simulink model "DCMGHILS"  (Simulink 7.9)
settings: Solver=ode4  StartTime=0.0  StopTime=inf  FixedStep=.1  RelTol=1e-3
StartFcn:
  | h=add_exec_event_listener('DCMGHILS/GUIScope','PostOutputs',@GUIScope);
values from neighbouring files (symbols this model uses):
  Manual = evalin('base','Manual')    [DCMicrogrid2.m]
libraries: simulink x24, opclib x3
settings Model: Creator=Don  LastModifiedBy=Microgrid_Project
settings DebuggingCC: FcnCallInpInsideContextMsg=Use local settings
settings GRTTargetCC: CombineOutputUpdateFcns=off  GRTInterface=on

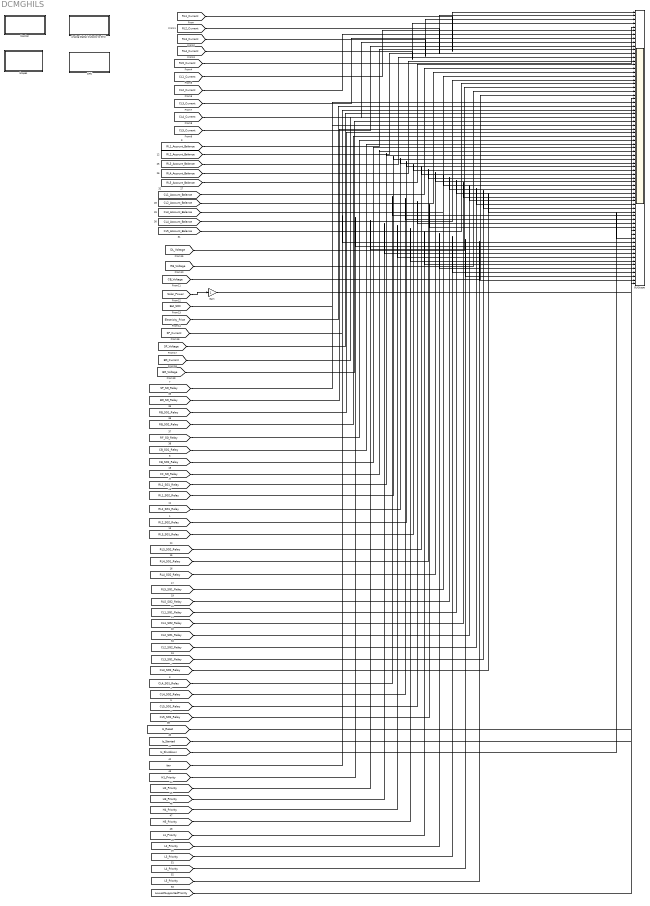
== system DCMGHILS ==
  Analog Digital Outputs to Grid : Subsystem
  GUIScope : Scope  NumInputPorts=73
      settings: YMin=-5~-5~-5~-5~-5~-5~-5~-5~-5~-5~-5~-5~-5~-5~-5~-5~-5~-5~-5~-5~-5~-5~-5~-5~-5~-5~-5~-5~-5~-5~-5~-5~-5~-5~-5~-5~-5~-5~-5~-5~-5~-5~-5~-5~-5~-5~-5~-5~-5~-5~-5~-5~-5~-5~-5~-5~-5~-5~-5~-5~-5~-5~-5~-5~-5~-5~-5~-5~-5~-5~-5~-5~-5  YMax=5~5~5~5~5~5~5~5~5~5~5~5~5~5~5~5~5~5~5~5~5~5~5~5~5~5~5~5~5~5~5~5~5~5~5~5~5~5~5~5~5~5~5~5~5~5~5~5~5~5~5~5~5~5~5~5~5~5~5~5~5~5~5~5~5~5~5~5~5~5~5~5~5  MaxDataPoints=10  SampleInput=on  SampleTime=.1
  Gain : Gain
  Monitor : Subsystem
  OPC : Subsystem
  Scopes : Subsystem
  wires:
  [Solar_Power] -> Gain/1
  [RL1_Current] -> GUIScope/1
  [RL2_Current] -> GUIScope/2
  [RL3_Current] -> GUIScope/3
  [RL4_Current] -> GUIScope/4
  [RL5_Current] -> GUIScope/5
  [CL1_Current] -> GUIScope/6
  [CL2_Current] -> GUIScope/7
  Gain/1 -> GUIScope/24
  [CL3_Current] -> GUIScope/8
  [CL4_Current] -> GUIScope/9
  [CL5_Current] -> GUIScope/10
  [RL1_Account_Balance] -> GUIScope/11
  [RL2_Account_Balance] -> GUIScope/12
  [RL3_Account_Balance] -> GUIScope/13
  [RL4_Account_Balance] -> GUIScope/14
  [RL5_Account_Balance] -> GUIScope/15
  [CL1_Account_Balance] -> GUIScope/16
  [CL2_Account_Balance] -> GUIScope/17
  [CL3_Account_Balance] -> GUIScope/18
  [CL4_Account_Balance] -> GUIScope/19
  [CL5_Account_Balance] -> GUIScope/20
  [DL_Voltage] -> GUIScope/21
  [RB_Voltage] -> GUIScope/22
  [CB_Voltage] -> GUIScope/23
  [Bat_SOC] -> GUIScope/25
  [Electricity_Price] -> GUIScope/26
  [SP_Current] -> GUIScope/27
  [SP_Voltage] -> GUIScope/28
  [BG_Current] -> GUIScope/29
  [BG_Voltage] -> GUIScope/30
  [SP_SG_Relay] -> GUIScope/31
  [BG_SG_Relay] -> GUIScope/32
  [RB_SG1_Relay] -> GUIScope/33
  [RB_SG2_Relay] -> GUIScope/34
  [RF_SG_Relay] -> GUIScope/35
  [CB_SG1_Relay] -> GUIScope/36
  [CB_SG2_Relay] -> GUIScope/37
  [CF_SG_Relay] -> GUIScope/38
  [RL1_SG1_Relay] -> GUIScope/39
  [RL1_SG2_Relay] -> GUIScope/40
  [RL2_SG1_Relay] -> GUIScope/41
  [RL2_SG2_Relay] -> GUIScope/42
  [RL3_SG1_Relay] -> GUIScope/43
  [RL3_SG2_Relay] -> GUIScope/44
  [RL4_SG1_Relay] -> GUIScope/45
  [RL4_SG2_Relay] -> GUIScope/46
  [RL5_SG1_Relay] -> GUIScope/47
  [RL5_SG2_Relay] -> GUIScope/48
  [CL1_SG1_Relay] -> GUIScope/49
  [CL1_SG2_Relay] -> GUIScope/50
  [CL2_SG1_Relay] -> GUIScope/51
  [CL2_SG2_Relay] -> GUIScope/52
  [CL3_SG1_Relay] -> GUIScope/53
  [CL3_SG2_Relay] -> GUIScope/54
  [CL4_SG1_Relay] -> GUIScope/55
  [CL4_SG2_Relay] -> GUIScope/56
  [CL5_SG1_Relay] -> GUIScope/57
  [CL5_SG2_Relay] -> GUIScope/58
  [iter] -> GUIScope/62
  [H1_Priority] -> GUIScope/63
  [H2_Priority] -> GUIScope/64
  [H3_Priority] -> GUIScope/65
  [H4_Priority] -> GUIScope/66
  [H5_Priority] -> GUIScope/67
  [L1_Priority] -> GUIScope/68
  [L2_Priority] -> GUIScope/69
  [L3_Priority] -> GUIScope/70
  [L4_Priority] -> GUIScope/71
  [L5_Priority] -> GUIScope/72
  [Is_Reset] -> GUIScope/59
  [Is_Started] -> GUIScope/60
  [Is_Shutdown] -> GUIScope/61
  [LowestSupportedPriority] -> GUIScope/73

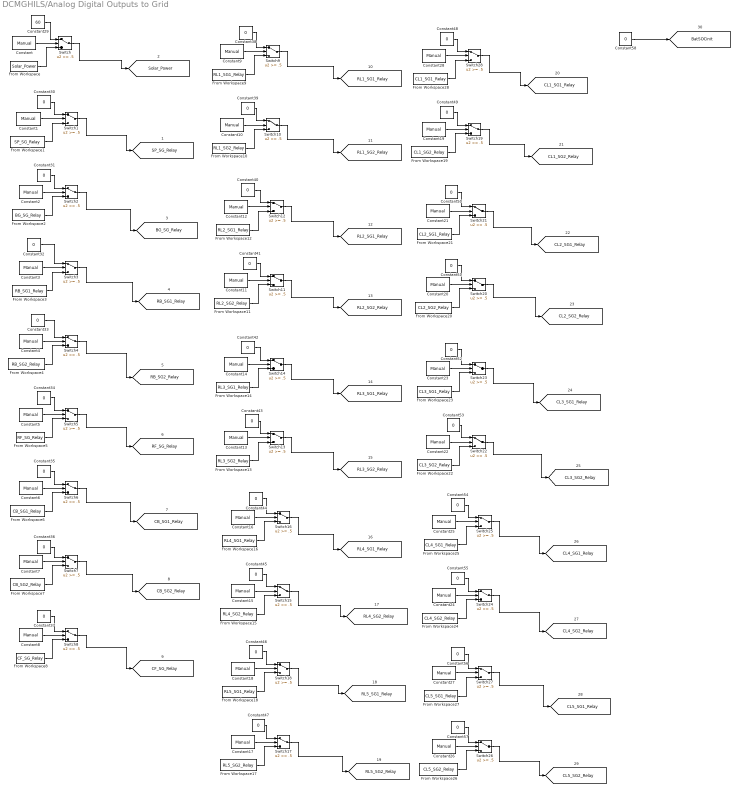
== system DCMGHILS/Analog Digital Outputs to Grid ==
  Constant{,1..28} (29 alike) : Constant  Value=Manual
  Constant29 : Constant  Value=60
  Constant{30..58} (29 alike) : Constant  Value=0
  From Workspace : FromWorkspace  VariableName=Solar_Power  SampleTime=0  Interpolate=off  OutputAfterFinalValue=Holding final value
  From Workspace1 : FromWorkspace  VariableName=SP_SG_Relay  SampleTime=0  Interpolate=off  OutputAfterFinalValue=Holding final value
  From Workspace10 : FromWorkspace  VariableName=RL1_SG2_Relay  SampleTime=0  Interpolate=off  OutputAfterFinalValue=Holding final value
  From Workspace11 : FromWorkspace  VariableName=RL2_SG2_Relay  SampleTime=0  Interpolate=off  OutputAfterFinalValue=Holding final value
  From Workspace12 : FromWorkspace  VariableName=RL2_SG1_Relay  SampleTime=0  Interpolate=off  OutputAfterFinalValue=Holding final value
  From Workspace13 : FromWorkspace  VariableName=RL3_SG2_Relay  SampleTime=0  Interpolate=off  OutputAfterFinalValue=Holding final value
  From Workspace14 : FromWorkspace  VariableName=RL3_SG1_Relay  SampleTime=0  Interpolate=off  OutputAfterFinalValue=Holding final value
  From Workspace15 : FromWorkspace  VariableName=RL4_SG2_Relay  SampleTime=0  Interpolate=off  OutputAfterFinalValue=Holding final value
  From Workspace16 : FromWorkspace  VariableName=RL4_SG1_Relay  SampleTime=0  Interpolate=off  OutputAfterFinalValue=Holding final value
  From Workspace17 : FromWorkspace  VariableName=RL5_SG2_Relay  SampleTime=0  Interpolate=off  OutputAfterFinalValue=Holding final value
  From Workspace18 : FromWorkspace  VariableName=RL5_SG1_Relay  SampleTime=0  Interpolate=off  OutputAfterFinalValue=Holding final value
  From Workspace19 : FromWorkspace  VariableName=CL1_SG2_Relay  SampleTime=0  Interpolate=off  OutputAfterFinalValue=Holding final value
  From Workspace2 : FromWorkspace  VariableName=BG_SG_Relay  SampleTime=0  Interpolate=off  OutputAfterFinalValue=Holding final value
  From Workspace20 : FromWorkspace  VariableName=CL2_SG2_Relay  SampleTime=0  Interpolate=off  OutputAfterFinalValue=Holding final value
  From Workspace21 : FromWorkspace  VariableName=CL2_SG1_Relay  SampleTime=0  Interpolate=off  OutputAfterFinalValue=Holding final value
  From Workspace22 : FromWorkspace  VariableName=CL3_SG2_Relay  SampleTime=0  Interpolate=off  OutputAfterFinalValue=Holding final value
  From Workspace23 : FromWorkspace  VariableName=CL3_SG1_Relay  SampleTime=0  Interpolate=off  OutputAfterFinalValue=Holding final value
  From Workspace24 : FromWorkspace  VariableName=CL4_SG2_Relay  SampleTime=0  Interpolate=off  OutputAfterFinalValue=Holding final value
  From Workspace25 : FromWorkspace  VariableName=CL4_SG1_Relay  SampleTime=0  Interpolate=off  OutputAfterFinalValue=Holding final value
  From Workspace26 : FromWorkspace  VariableName=CL5_SG2_Relay  SampleTime=0  Interpolate=off  OutputAfterFinalValue=Holding final value
  From Workspace27 : FromWorkspace  VariableName=CL5_SG1_Relay  SampleTime=0  Interpolate=off  OutputAfterFinalValue=Holding final value
  From Workspace28 : FromWorkspace  VariableName=CL1_SG1_Relay  SampleTime=0  Interpolate=off  OutputAfterFinalValue=Holding final value
  From Workspace3 : FromWorkspace  VariableName=RB_SG1_Relay  SampleTime=0  Interpolate=off  OutputAfterFinalValue=Holding final value
  From Workspace4 : FromWorkspace  VariableName=RB_SG2_Relay  SampleTime=0  Interpolate=off  OutputAfterFinalValue=Holding final value
  From Workspace5 : FromWorkspace  VariableName=RF_SG_Relay  SampleTime=0  Interpolate=off  OutputAfterFinalValue=Holding final value
  From Workspace6 : FromWorkspace  VariableName=CB_SG1_Relay  SampleTime=0  Interpolate=off  OutputAfterFinalValue=Holding final value
  From Workspace7 : FromWorkspace  VariableName=CB_SG2_Relay  SampleTime=0  Interpolate=off  OutputAfterFinalValue=Holding final value
  From Workspace8 : FromWorkspace  VariableName=CF_SG_Relay  SampleTime=0  Interpolate=off  OutputAfterFinalValue=Holding final value
  From Workspace9 : FromWorkspace  VariableName=RL1_SG1_Relay  SampleTime=0  Interpolate=off  OutputAfterFinalValue=Holding final value
  Switch{,1..28} (29 alike) : Switch  Threshold=.5
  tag scope: BG_SG_Relay=global, BatSOCinit=global, CB_SG1_Relay=global, CB_SG2_Relay=global, CF_SG_Relay=global, CL1_SG1_Relay=global, CL1_SG2_Relay=global, CL2_SG1_Relay=global, CL2_SG2_Relay=global, CL3_SG1_Relay=global, CL3_SG2_Relay=global, CL4_SG1_Relay=global, CL4_SG2_Relay=global, CL5_SG1_Relay=global, CL5_SG2_Relay=global, RB_SG1_Relay=global, RB_SG2_Relay=global, RF_SG_Relay=global, RL1_SG1_Relay=global, RL1_SG2_Relay=global, RL2_SG1_Relay=global, RL2_SG2_Relay=global, RL3_SG1_Relay=global, RL3_SG2_Relay=global, RL4_SG1_Relay=global, RL4_SG2_Relay=global, RL5_SG1_Relay=global, RL5_SG2_Relay=global, SP_SG_Relay=global, Solar_Power=global
  wires:
  Constant/1 -> Switch/2
  From Workspace/1 -> Switch/3
  Constant29/1 -> Switch/1
  Switch/1 -> [Solar_Power]
  Constant1/1 -> Switch1/2
  From Workspace1/1 -> Switch1/3
  Constant30/1 -> Switch1/1
  Switch1/1 -> [SP_SG_Relay]
  Constant2/1 -> Switch2/2
  From Workspace2/1 -> Switch2/3
  Constant31/1 -> Switch2/1
  Switch2/1 -> [BG_SG_Relay]
  Constant3/1 -> Switch3/2
  From Workspace3/1 -> Switch3/3
  Constant32/1 -> Switch3/1
  Switch3/1 -> [RB_SG1_Relay]
  Constant4/1 -> Switch4/2
  From Workspace4/1 -> Switch4/3
  Constant33/1 -> Switch4/1
  Switch4/1 -> [RB_SG2_Relay]
  Constant5/1 -> Switch5/2
  From Workspace5/1 -> Switch5/3
  Constant34/1 -> Switch5/1
  Switch5/1 -> [RF_SG_Relay]
  Constant6/1 -> Switch6/2
  From Workspace6/1 -> Switch6/3
  Constant35/1 -> Switch6/1
  Switch6/1 -> [CB_SG1_Relay]
  Constant7/1 -> Switch7/2
  From Workspace7/1 -> Switch7/3
  Constant36/1 -> Switch7/1
  Switch7/1 -> [CB_SG2_Relay]
  Constant8/1 -> Switch8/2
  From Workspace8/1 -> Switch8/3
  Constant37/1 -> Switch8/1
  Switch8/1 -> [CF_SG_Relay]
  Constant9/1 -> Switch9/2
  From Workspace9/1 -> Switch9/3
  Constant38/1 -> Switch9/1
  Switch9/1 -> [RL1_SG1_Relay]
  Constant10/1 -> Switch10/2
  From Workspace10/1 -> Switch10/3
  Constant39/1 -> Switch10/1
  Switch10/1 -> [RL1_SG2_Relay]
  Constant12/1 -> Switch12/2
  From Workspace12/1 -> Switch12/3
  Constant40/1 -> Switch12/1
  Switch12/1 -> [RL2_SG1_Relay]
  Constant11/1 -> Switch11/2
  From Workspace11/1 -> Switch11/3
  Constant41/1 -> Switch11/1
  Switch11/1 -> [RL2_SG2_Relay]
  Constant14/1 -> Switch14/2
  From Workspace14/1 -> Switch14/3
  Constant42/1 -> Switch14/1
  Switch14/1 -> [RL3_SG1_Relay]
  Constant13/1 -> Switch13/2
  From Workspace13/1 -> Switch13/3
  Constant43/1 -> Switch13/1
  Switch13/1 -> [RL3_SG2_Relay]
  Constant16/1 -> Switch16/2
  From Workspace16/1 -> Switch16/3
  Constant44/1 -> Switch16/1
  Switch16/1 -> [RL4_SG1_Relay]
  Constant15/1 -> Switch15/2
  From Workspace15/1 -> Switch15/3
  Constant45/1 -> Switch15/1
  Switch15/1 -> [RL4_SG2_Relay]
  Constant18/1 -> Switch18/2
  From Workspace18/1 -> Switch18/3
  Constant46/1 -> Switch18/1
  Switch18/1 -> [RL5_SG1_Relay]
  Constant17/1 -> Switch17/2
  From Workspace17/1 -> Switch17/3
  Constant47/1 -> Switch17/1
  Switch17/1 -> [RL5_SG2_Relay]
  Constant28/1 -> Switch28/2
  From Workspace28/1 -> Switch28/3
  Constant48/1 -> Switch28/1
  Switch28/1 -> [CL1_SG1_Relay]
  Constant19/1 -> Switch19/2
  From Workspace19/1 -> Switch19/3
  Constant49/1 -> Switch19/1
  Switch19/1 -> [CL1_SG2_Relay]
  Constant21/1 -> Switch21/2
  From Workspace21/1 -> Switch21/3
  Constant50/1 -> Switch21/1
  Switch21/1 -> [CL2_SG1_Relay]
  Constant20/1 -> Switch20/2
  From Workspace20/1 -> Switch20/3
  Constant51/1 -> Switch20/1
  Switch20/1 -> [CL2_SG2_Relay]
  Constant23/1 -> Switch23/2
  From Workspace23/1 -> Switch23/3
  Constant52/1 -> Switch23/1
  Switch23/1 -> [CL3_SG1_Relay]
  Constant22/1 -> Switch22/2
  From Workspace22/1 -> Switch22/3
  Constant53/1 -> Switch22/1
  Switch22/1 -> [CL3_SG2_Relay]
  Constant25/1 -> Switch25/2
  From Workspace25/1 -> Switch25/3
  Constant54/1 -> Switch25/1
  Switch25/1 -> [CL4_SG1_Relay]
  Constant24/1 -> Switch24/2
  From Workspace24/1 -> Switch24/3
  Constant55/1 -> Switch24/1
  Switch24/1 -> [CL4_SG2_Relay]
  Constant27/1 -> Switch27/2
  From Workspace27/1 -> Switch27/3
  Constant56/1 -> Switch27/1
  Switch27/1 -> [CL5_SG1_Relay]
  Constant26/1 -> Switch26/2
  From Workspace26/1 -> Switch26/3
  Constant57/1 -> Switch26/1
  Switch26/1 -> [CL5_SG2_Relay]
  Constant58/1 -> [BatSOCinit]

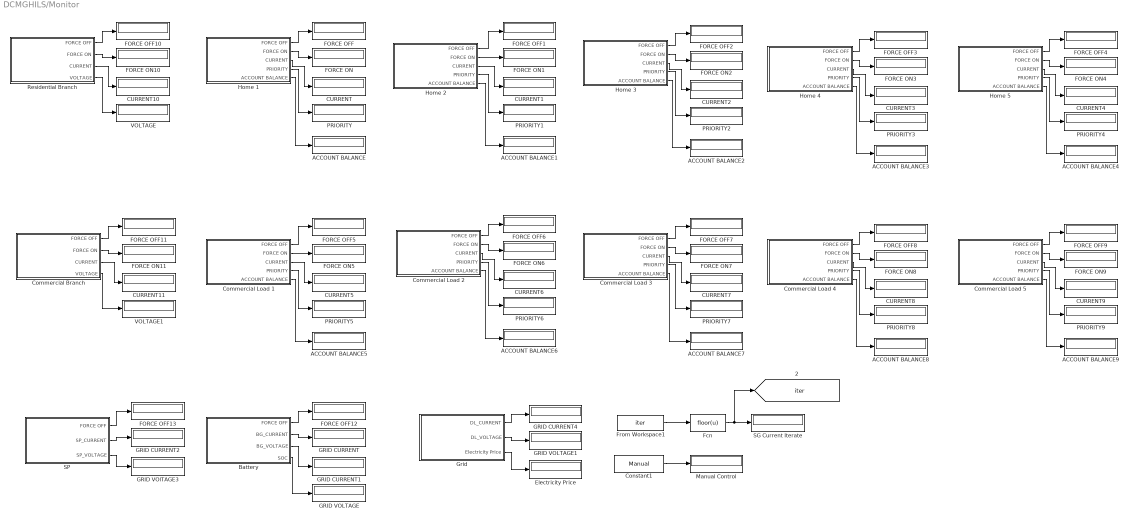
== system DCMGHILS/Monitor ==
  ACCOUNT BALANCE{,1..9} (10 alike) : Display
  Battery : Subsystem
  CURRENT{,1..11} (12 alike) : Display
  Commercial Branch : Subsystem
  Commercial Load 1 : Subsystem
  Commercial Load 2 : Subsystem
  Commercial Load 3 : Subsystem
  Commercial Load 4 : Subsystem
  Commercial Load 5 : Subsystem
  Constant1 : Constant  Value=Manual
  Electricity Price : Display
  FORCE OFF{,1..13} (14 alike) : Display
  FORCE ON{,1..11} (12 alike) : Display
  Fcn : Fcn  Expr=floor(u)
  From Workspace1 : FromWorkspace  VariableName=iter  SampleTime=0
  GRID CURRENT{,1..2,4} (4 alike) : Display
  GRID VOLTAGE : Display
  GRID VOLTAGE1 : Display
  GRID VOlTAGE3 : Display
  Grid : Subsystem
  Home 1 : Subsystem
  Home 2 : Subsystem
  Home 3 : Subsystem
  Home 4 : Subsystem
  Home 5 : Subsystem
  Manual Control : Display
  PRIORITY{,1..9} (10 alike) : Display
  Residential Branch : Subsystem
  SG Current Iterate : Display
  SP : Subsystem
  VOLTAGE : Display
  VOLTAGE1 : Display
  tag scope: iter=global
  wires:
  Home 1/1(FORCE OFF) -> FORCE OFF/1
  Home 1/2(FORCE ON) -> FORCE ON/1
  Home 1/3(CURRENT) -> CURRENT/1
  Home 1/4(PRIORITY) -> PRIORITY/1
  Home 1/5(ACCOUNT BALANCE) -> ACCOUNT BALANCE/1
  Home 2/1(FORCE OFF) -> FORCE OFF1/1
  Home 2/2(FORCE ON) -> FORCE ON1/1
  Home 2/3(CURRENT) -> CURRENT1/1
  Home 2/4(PRIORITY) -> PRIORITY1/1
  Home 2/5(ACCOUNT BALANCE) -> ACCOUNT BALANCE1/1
  Home 3/1(FORCE OFF) -> FORCE OFF2/1
  Home 3/2(FORCE ON) -> FORCE ON2/1
  Home 3/3(CURRENT) -> CURRENT2/1
  Home 3/4(PRIORITY) -> PRIORITY2/1
  Home 3/5(ACCOUNT BALANCE) -> ACCOUNT BALANCE2/1
  Home 4/1(FORCE OFF) -> FORCE OFF3/1
  Home 4/2(FORCE ON) -> FORCE ON3/1
  Home 4/3(CURRENT) -> CURRENT3/1
  Home 4/4(PRIORITY) -> PRIORITY3/1
  Home 4/5(ACCOUNT BALANCE) -> ACCOUNT BALANCE3/1
  Home 5/1(FORCE OFF) -> FORCE OFF4/1
  Home 5/2(FORCE ON) -> FORCE ON4/1
  Home 5/3(CURRENT) -> CURRENT4/1
  Home 5/4(PRIORITY) -> PRIORITY4/1
  Home 5/5(ACCOUNT BALANCE) -> ACCOUNT BALANCE4/1
  Commercial Load 1/1(FORCE OFF) -> FORCE OFF5/1
  Commercial Load 1/2(FORCE ON) -> FORCE ON5/1
  Commercial Load 1/3(CURRENT) -> CURRENT5/1
  Commercial Load 1/4(PRIORITY) -> PRIORITY5/1
  Commercial Load 1/5(ACCOUNT BALANCE) -> ACCOUNT BALANCE5/1
  Commercial Load 2/1(FORCE OFF) -> FORCE OFF6/1
  Commercial Load 2/2(FORCE ON) -> FORCE ON6/1
  Commercial Load 2/3(CURRENT) -> CURRENT6/1
  Commercial Load 2/4(PRIORITY) -> PRIORITY6/1
  Commercial Load 2/5(ACCOUNT BALANCE) -> ACCOUNT BALANCE6/1
  Commercial Load 3/1(FORCE OFF) -> FORCE OFF7/1
  Commercial Load 3/2(FORCE ON) -> FORCE ON7/1
  Commercial Load 3/3(CURRENT) -> CURRENT7/1
  Commercial Load 3/4(PRIORITY) -> PRIORITY7/1
  Commercial Load 3/5(ACCOUNT BALANCE) -> ACCOUNT BALANCE7/1
  Commercial Load 4/1(FORCE OFF) -> FORCE OFF8/1
  Commercial Load 4/2(FORCE ON) -> FORCE ON8/1
  Commercial Load 4/3(CURRENT) -> CURRENT8/1
  Commercial Load 4/4(PRIORITY) -> PRIORITY8/1
  Commercial Load 4/5(ACCOUNT BALANCE) -> ACCOUNT BALANCE8/1
  Commercial Load 5/1(FORCE OFF) -> FORCE OFF9/1
  Commercial Load 5/2(FORCE ON) -> FORCE ON9/1
  Commercial Load 5/3(CURRENT) -> CURRENT9/1
  Commercial Load 5/4(PRIORITY) -> PRIORITY9/1
  Commercial Load 5/5(ACCOUNT BALANCE) -> ACCOUNT BALANCE9/1
  Residential Branch/1(FORCE OFF) -> FORCE OFF10/1
  Residential Branch/2(FORCE ON) -> FORCE ON10/1
  Residential Branch/3(CURRENT) -> CURRENT10/1
  Residential Branch/4(VOLTAGE) -> VOLTAGE/1
  Commercial Branch/1(FORCE OFF) -> FORCE OFF11/1
  Commercial Branch/2(FORCE ON) -> FORCE ON11/1
  Commercial Branch/3(CURRENT) -> CURRENT11/1
  Commercial Branch/4(VOLTAGE) -> VOLTAGE1/1
  Battery/1(FORCE OFF) -> FORCE OFF12/1
  Battery/2(BG_CURRENT) -> GRID CURRENT/1
  Battery/3(BG_VOLTAGE) -> GRID CURRENT1/1
  Battery/4(SOC) -> GRID VOLTAGE/1
  Grid/1(DL_CURRENT) -> GRID CURRENT4/1
  Grid/2(DL_VOLTAGE) -> GRID VOLTAGE1/1
  Grid/3(Electricity Price) -> Electricity Price/1
  Constant1/1 -> Manual Control/1
  SP/1(FORCE OFF) -> FORCE OFF13/1
  SP/2(SP_CURRENT) -> GRID CURRENT2/1
  SP/3(SP_VOLTAGE) -> GRID VOlTAGE3/1
  From Workspace1/1 -> Fcn/1
  Fcn/1 -> SG Current Iterate/1, [iter]

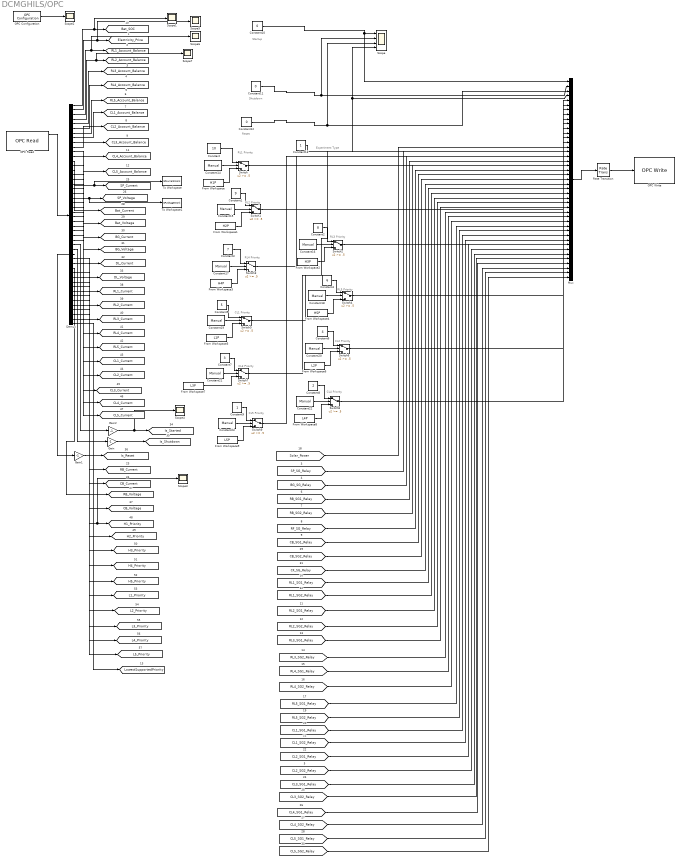
== system DCMGHILS/OPC ==
  note: Startup
  note: Experiment Type
  note: Shutdown
  note: Reset
  note: RL1 Priority
  note: RL2 Priority
  note: RL3 Priority
  note: RL4 Priority
  note: CL1 Priority
  note: CL2 Priority
  note: CL3 Priority
  note: CL4 Priority
  note: CL5 Priority
  note: RL5 Priority
  Constant : Constant  Value=10
  Constant1 : Constant  Value=9
  Constant10 : Constant  Value=0
  Constant11 : Constant  Value=0
  Constant12 : Constant  Value=0
  Constant13 : Constant
  Constant{14..23} (10 alike) : Constant  Value=Manual
  Constant2 : Constant  Value=8
  Constant3 : Constant  Value=7
  Constant4 : Constant  Value=6
  Constant5 : Constant  Value=5
  Constant6 : Constant  Value=4
  Constant7 : Constant  Value=3
  Constant8 : Constant  Value=2
  Constant9 : Constant
  Demux : Demux  Outputs=48
  From Workspace : FromWorkspace  VariableName=H1P  SampleTime=0  Interpolate=off  OutputAfterFinalValue=Holding final value
  From Workspace1 : FromWorkspace  VariableName=H2P  SampleTime=0  Interpolate=off  OutputAfterFinalValue=Holding final value
  From Workspace2 : FromWorkspace  VariableName=H3P  SampleTime=0  Interpolate=off  OutputAfterFinalValue=Holding final value
  From Workspace3 : FromWorkspace  VariableName=H4P  SampleTime=0  Interpolate=off  OutputAfterFinalValue=Holding final value
  From Workspace4 : FromWorkspace  VariableName=H5P  SampleTime=0  Interpolate=off  OutputAfterFinalValue=Holding final value
  From Workspace5 : FromWorkspace  VariableName=L1P  SampleTime=0  Interpolate=off  OutputAfterFinalValue=Holding final value
  From Workspace6 : FromWorkspace  VariableName=L2P  SampleTime=0  Interpolate=off  OutputAfterFinalValue=Holding final value
  From Workspace7 : FromWorkspace  VariableName=L3P  SampleTime=0  Interpolate=off  OutputAfterFinalValue=Holding final value
  From Workspace8 : FromWorkspace  VariableName=L4P  SampleTime=0  Interpolate=off  OutputAfterFinalValue=Holding final value
  From Workspace9 : FromWorkspace  VariableName=L5P  SampleTime=0  Interpolate=off  OutputAfterFinalValue=Holding final value
  Gain : Gain  Gain=-1
  Gain1 : Gain  Gain=-1
  Gain2 : Gain  Gain=-1
  Mux : Mux  Inputs=43
  OPC Configuration : opclib/OPC Configuration  opcServers=localhost/FactoryTalk Gateway/10  errMissingItems=Error  errReadWrite=Warn  errShutdown=Error  errRTViolation=Warn  rtEnable=on  speedup=1  showLatency=on  beingUsed=on
  OPC Read : opclib/OPC Read  serverHost=localhost  serverID=FactoryTalk Gateway  itemIDs=[smartgrid]Batterysoc, [smartgrid]DCMicroGridpowerRate, [smartgrid]House01accountBalance, [smartgrid]House02accountBalance, [smartgrid]House03accountBalance, [smartgrid]House04accountBalance, [smartgrid]House05accountBalance, [smartgrid]Load01accountBalance, [smartgrid]Load02accountBalance, [smartgrid]Load03accountBalance, [smartgrid]Load04accountBalance, [smartgrid]Load05accountBalance, [smartgrid]SolarPanelcurrent, [smartgrid]SolarPanelvoltage, [smartgrid]BatterybattCurrent, [smartgrid]BatterybattVoltage, [smartgrid]BatterygridCurrent, [smartgrid]BatterygridVoltage, [smartgrid]Loadscurrent, [smartgrid]Loadsvoltage, [smartgrid]House01current, [smartgrid]House02current, [smartgrid]House03current, [smartgrid]House04current, [smartgrid]House05current, [smartgrid]Load01current, [smartgrid]Load02current, [smartgrid]Load03current, [smartgrid]Load04current, [smartgrid]Load05current, [smartgrid]DCMicroGridisStarted, [smartgrid]DCMicroGridisShutdown, [smartgrid]DCMicroGridResetEventSuccess, [smartgrid]Rescurrent, [smartgrid]Commcurrent, [smartgrid]Resvoltage, [smartgrid]Commvoltage, [smartgrid]House01priority, [smartgrid]House02priority, [smartgrid]House03priority, [smartgrid]House04priority, [smartgrid]House05priority, [smartgrid]Load01priority, [smartgrid]Load02priority, [smartgrid]Load03priority, [smartgrid]Load04priority, [smartgrid]Load05priority, [smartgrid]DCMicroGridlowestSupportedPriority  readMode=Asynchronous (device)  dataType=double  updateRate=0.1  showQual=on  showTS=on  tsMode=Seconds since start
  OPC Write : opclib/OPC Write  serverHost=localhost  serverID=FactoryTalk Gateway  itemIDs=[smartgrid]DCMicroGridreqStartup, [smartgrid]DCMicroGridreqShutdown, [smartgrid]DCMicroGridreqReset, [smartgrid]DCMicroGridisSimulating, [smartgrid]House01priority, [smartgrid]House02priority, [smartgrid]House03priority, [smartgrid]House04priority, [smartgrid]House05priority, [smartgrid]Load01priority, [smartgrid]Load02priority, [smartgrid]Load03priority, [smartgrid]Load04priority, [smartgrid]Load05priority, [smartgrid]Solar_Power, [smartgrid]SP_SG_Relay, [smartgrid]BG_SG_Relay, [smartgrid]RB_SG1_Relay, [smartgrid]RB_SG2_Relay, [smartgrid]RF_SG_Relay, [smartgrid]CB_SG1_Relay, [smartgrid]CB_SG2_Relay, [smartgrid]CF_SG_Relay, [smartgrid]RL1_SG1_Relay, [smartgrid]RL1_SG2_Relay, [smartgrid]RL2_SG1_Relay, [smartgrid]RL2_SG2_Relay, [smartgrid]RL3_SG1_Relay, [smartgrid]RL3_SG2_Relay, [smartgrid]RL4_SG1_Relay, [smartgrid]RL4_SG2_Relay, [smartgrid]RL5_SG1_Relay, [smartgrid]RL5_SG2_Relay, [smartgrid]CL1_SG1_Relay, [smartgrid]CL1_SG2_Relay, [smartgrid]CL2_SG1_Relay, [smartgrid]CL2_SG2_Relay, [smartgrid]CL3_SG1_Relay, [smartgrid]CL3_SG2_Relay, [smartgrid]CL4_SG1_Relay, [smartgrid]CL4_SG2_Relay, [smartgrid]CL5_SG1_Relay, [smartgrid]CL5_SG2_Relay  writeMode=Asynchronous  updateRate=0.1
  Rate Transition : RateTransition  OutPortSampleTime=.1
  Scope : Scope  NumInputPorts=4
      settings: TimeRange=50  YMin=-1~-1~1~1  YMax=1~1~1~1  SaveName=ScopeData3
  Scope{1..7} (7 alike) : Scope
      Scope1 settings: TimeRange=50  YMin=-0.8  YMax=0.05  SaveName=ScopeData5
      Scope2 settings: TimeRange=50  YMin=-0.8  YMax=0.05  SaveName=ScopeData4
      Scope3 settings: TimeRange=50  YMin=-0.8  YMax=0.05  SaveName=ScopeData7
      Scope4 settings: TimeRange=50  YMin=0.000113985  YMax=0.000125983  SaveName=ScopeData6
      Scope5 settings: TimeRange=50  YMin=100  YMax=100  SaveName=ScopeData8
      Scope6 settings: TimeRange=50  YMin=125  YMax=125  SaveName=ScopeData9
      Scope7 settings: TimeRange=50  YMin=1111  YMax=1111  SaveName=ScopeData10
  Switch{,1..9} (10 alike) : Switch  Threshold=.5
  To Workspace : ToWorkspace  VariableName=SPcurrentWork  SampleTime=-1
  To Workspace1 : ToWorkspace  VariableName=SPvoltageWork  SampleTime=-1
  tag scope: BG_Current=global, BG_Voltage=global, Bat_Current=global, Bat_SOC=global, Bat_Voltage=global, CB_Current=global, CB_Voltage=global, CL1_Account_Balance=global, CL1_Current=global, CL2_Account_Balance=global, CL2_Current=global, CL3_Account_Balance=global, CL3_Current=global, CL4_Account_Balance=global, CL4_Current=global, CL5_Account_Balance=global, CL5_Current=global, DL_Current=global, DL_Voltage=global, Electricity_Price=global, H1_Priority=global, H2_Priority=global, H3_Priority=global, H4_Priority=global, H5_Priority=global, Is_Reset=global, Is_Shutdown=global, Is_Started=global, L1_Priority=global, L2_Priority=global, L3_Priority=global, L4_Priority=global, L5_Priority=global, LowestSupportedPriority=global, RB_Current=global, RB_Voltage=global, RL1_Account_Balance=global, RL1_Current=global, RL2_Account_Balance=global, RL2_Current=global, RL3_Account_Balance=global, RL3_Current=global, RL4_Account_Balance=global, RL4_Current=global, RL5_Account_Balance=global, RL5_Current=global, SP_Current=global, SP_Voltage=global
  wires:
  OPC Configuration/1 -> Scope2/1
  OPC Read/1 -> Demux/1
  Demux/1 -> [Bat_SOC], Scope1/1
  Demux/2 -> [Electricity_Price], Scope5/1
  Demux/3 -> [RL1_Account_Balance], Scope6/1
  Demux/4 -> [RL2_Account_Balance], Scope7/1
  Demux/5 -> [RL3_Account_Balance]
  Demux/6 -> [RL4_Account_Balance]
  Demux/7 -> [RL5_Account_Balance]
  Demux/8 -> [CL1_Account_Balance]
  Demux/9 -> [CL2_Account_Balance]
  Demux/10 -> [CL3_Account_Balance]
  Demux/11 -> [CL4_Account_Balance]
  Demux/12 -> [CL5_Account_Balance]
  Demux/13 -> [SP_Current], To Workspace/1
  Demux/14 -> [SP_Voltage], To Workspace1/1
  Demux/15 -> [Bat_Current]
  Demux/16 -> [Bat_Voltage]
  Demux/17 -> [BG_Current]
  Demux/18 -> [BG_Voltage]
  Demux/19 -> [DL_Current]
  Demux/20 -> [DL_Voltage]
  Demux/21 -> [RL1_Current]
  Demux/22 -> [RL2_Current]
  Demux/23 -> [RL3_Current]
  Demux/24 -> [RL4_Current]
  Demux/25 -> [RL5_Current]
  Demux/26 -> [CL1_Current]
  Demux/27 -> [CL2_Current]
  Demux/28 -> [CL3_Current]
  Demux/29 -> [CL4_Current]
  Demux/30 -> [CL5_Current]
  Demux/31 -> Gain2/1
  Demux/32 -> Gain/1
  Demux/33 -> Gain1/1
  Constant11/1 -> Mux/2, Scope/2
  Constant12/1 -> Scope/3, Mux/3
  Constant13/1 -> Scope/4, Mux/4
  Constant10/1 -> Mux/1, Scope/1
  Mux/1 -> Rate Transition/1
  Rate Transition/1 -> OPC Write/1
  [Solar_Power] -> Mux/15
  [SP_SG_Relay] -> Mux/16
  [BG_SG_Relay] -> Mux/17
  [RB_SG1_Relay] -> Mux/18
  [RB_SG2_Relay] -> Mux/19
  [RF_SG_Relay] -> Mux/20
  [CB_SG1_Relay] -> Mux/21
  [CB_SG2_Relay] -> Mux/22
  [CF_SG_Relay] -> Mux/23
  [RL1_SG1_Relay] -> Mux/24
  [RL1_SG2_Relay] -> Mux/25
  [RL2_SG1_Relay] -> Mux/26
  [RL2_SG2_Relay] -> Mux/27
  [RL3_SG1_Relay] -> Mux/28
  [RL3_SG2_Relay] -> Mux/29
  [RL4_SG1_Relay] -> Mux/30
  [RL4_SG2_Relay] -> Mux/31
  [RL5_SG1_Relay] -> Mux/32
  [RL5_SG2_Relay] -> Mux/33
  [CL1_SG1_Relay] -> Mux/34
  [CL1_SG2_Relay] -> Mux/35
  [CL2_SG1_Relay] -> Mux/36
  [CL2_SG2_Relay] -> Mux/37
  [CL3_SG1_Relay] -> Mux/38
  [CL3_SG2_Relay] -> Mux/39
  [CL4_SG1_Relay] -> Mux/40
  [CL4_SG2_Relay] -> Mux/41
  [CL5_SG1_Relay] -> Mux/42
  [CL5_SG2_Relay] -> Mux/43
  Demux/34 -> [RB_Current]
  Demux/35 -> [CB_Current]
  Demux/36 -> [RB_Voltage]
  Demux/37 -> [CB_Voltage]
  Gain/1 -> [Is_Shutdown]
  Gain1/1 -> [Is_Reset]
  Gain2/1 -> [Is_Started], Scope4/1
  Constant14/1 -> Switch/2
  From Workspace/1 -> Switch/3
  Constant/1 -> Switch/1
  Switch/1 -> Mux/5
  Constant15/1 -> Switch1/2
  From Workspace1/1 -> Switch1/3
  Constant1/1 -> Switch1/1
  Switch1/1 -> Mux/6
  Constant16/1 -> Switch2/2
  From Workspace2/1 -> Switch2/3
  Constant2/1 -> Switch2/1
  Switch2/1 -> Mux/7
  Constant17/1 -> Switch3/2
  From Workspace3/1 -> Switch3/3
  Constant3/1 -> Switch3/1
  Switch3/1 -> Mux/8
  Constant18/1 -> Switch4/2
  From Workspace4/1 -> Switch4/3
  Constant4/1 -> Switch4/1
  Switch4/1 -> Mux/9
  Constant19/1 -> Switch5/2
  From Workspace5/1 -> Switch5/3
  Constant5/1 -> Switch5/1
  Switch5/1 -> Mux/10
  Constant20/1 -> Switch6/2
  From Workspace6/1 -> Switch6/3
  Constant6/1 -> Switch6/1
  Switch6/1 -> Mux/11
  Constant21/1 -> Switch7/2
  From Workspace7/1 -> Switch7/3
  Constant7/1 -> Switch7/1
  Switch7/1 -> Mux/12
  Constant22/1 -> Switch8/2
  From Workspace8/1 -> Switch8/3
  Constant8/1 -> Switch8/1
  Switch8/1 -> Mux/13
  Constant23/1 -> Switch9/2
  From Workspace9/1 -> Switch9/3
  Constant9/1 -> Switch9/1
  Switch9/1 -> Mux/14
  Demux/38 -> [H1_Priority], Scope3/1
  Demux/39 -> [H2_Priority]
  Demux/40 -> [H3_Priority]
  Demux/41 -> [H4_Priority]
  Demux/42 -> [H5_Priority]
  Demux/43 -> [L1_Priority]
  Demux/44 -> [L2_Priority]
  Demux/45 -> [L3_Priority]
  Demux/46 -> [L4_Priority]
  Demux/47 -> [L5_Priority]
  Demux/48 -> [LowestSupportedPriority]

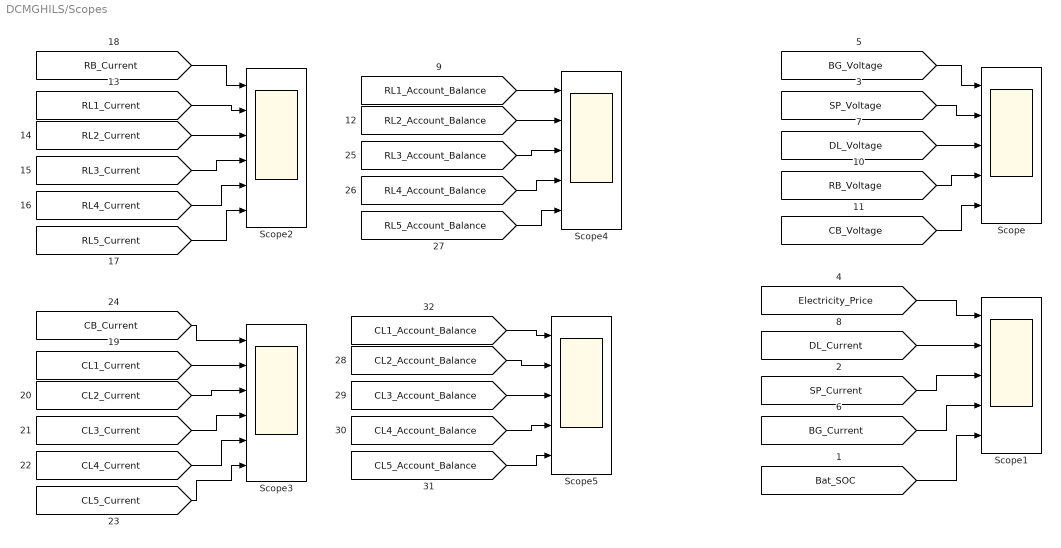
== system DCMGHILS/Scopes ==
  Scope{,1,4..5} (4 alike) : Scope  NumInputPorts=5
      Scope settings: YMin=11.4~0~0~0~0  YMax=12.6~12~12~12~12  SaveName=ScopeData2
      Scope1 settings: YMin=100~1.075~1.075~0.00011959~5.79821  YMax=100~1.325~1.325~0.00011967~5.79821  SaveName=ScopeData21
      Scope4 settings: YMin=26.368~26.701~26.41~26.701~26.399  YMax=26.374~26.708~26.416~26.708~26.406  SaveName=ScopeData24
      Scope5 settings: YMin=23.494~23.481~23.445~23.4615~15  YMax=23.498~23.485~23.449~23.4655~15  SaveName=ScopeData25
  Scope2 : Scope  NumInputPorts=6
      settings: YMin=5.55112e-17~1.38778e-17~1.38778e-17~1.38778e-17~1.38778e-17~1.38778e-17  YMax=1.4~0.25~0.25~0.25~0.25~0.25  SaveName=ScopeData22
  Scope3 : Scope  NumInputPorts=6
      settings: YMin=2.48833~0.497637~0.497637~0.497664~0.497637~0.497637  YMax=2.48833~0.497637~0.497637~0.497664~0.497637~0.497637  SaveName=ScopeData23
  wires:
  [RB_Current] -> Scope2/1
  [RL1_Current] -> Scope2/2
  [RL2_Current] -> Scope2/3
  [RL3_Current] -> Scope2/4
  [RL4_Current] -> Scope2/5
  [RL5_Current] -> Scope2/6
  [BG_Voltage] -> Scope/1
  [SP_Voltage] -> Scope/2
  [DL_Voltage] -> Scope/3
  [RB_Voltage] -> Scope/4
  [CB_Voltage] -> Scope/5
  [Electricity_Price] -> Scope1/1
  [DL_Current] -> Scope1/2
  [SP_Current] -> Scope1/3
  [BG_Current] -> Scope1/4
  [Bat_SOC] -> Scope1/5
  [CB_Current] -> Scope3/1
  [CL1_Current] -> Scope3/2
  [CL2_Current] -> Scope3/3
  [CL3_Current] -> Scope3/4
  [CL4_Current] -> Scope3/5
  [CL5_Current] -> Scope3/6
  [RL1_Account_Balance] -> Scope4/1
  [RL2_Account_Balance] -> Scope4/2
  [RL3_Account_Balance] -> Scope4/3
  [RL4_Account_Balance] -> Scope4/4
  [RL5_Account_Balance] -> Scope4/5
  [CL1_Account_Balance] -> Scope5/1
  [CL2_Account_Balance] -> Scope5/2
  [CL3_Account_Balance] -> Scope5/3
  [CL4_Account_Balance] -> Scope5/4
  [CL5_Account_Balance] -> Scope5/5

== system DCMGHILS/Monitor/Battery ==
  FORCE OFF : Outport
  BG_CURRENT : Outport  Port=2
  BG_VOLTAGE : Outport  Port=3
  SOC : Outport  Port=4
  wires:
  [BG_SG_Relay] -> FORCE OFF/1
  [BG_Current] -> BG_CURRENT/1
  [BG_Voltage] -> BG_VOLTAGE/1
  [Bat_SOC] -> SOC/1

== system DCMGHILS/Monitor/Commercial Branch ==
  Add : Sum
  Compare To Constant : simulink/Logic and Bit Operations/Compare To Constant  relop===  const=0  OutDataTypeStr=uint8
  Compare To Constant1 : simulink/Logic and Bit Operations/Compare To Constant  relop===  const=2  OutDataTypeStr=uint8
  FORCE OFF : Outport
  FORCE ON : Outport  Port=2
  CURRENT : Outport  Port=3
  VOLTAGE : Outport  Port=4
  wires:
  [CB_SG2_Relay] -> Compare To Constant/1, FORCE ON/1
  [CB_SG1_Relay] -> Add/1
  Compare To Constant/1 -> Add/2
  Add/1 -> Compare To Constant1/1
  Compare To Constant1/1 -> FORCE OFF/1
  [CB_Current] -> CURRENT/1
  [CB_Voltage] -> VOLTAGE/1

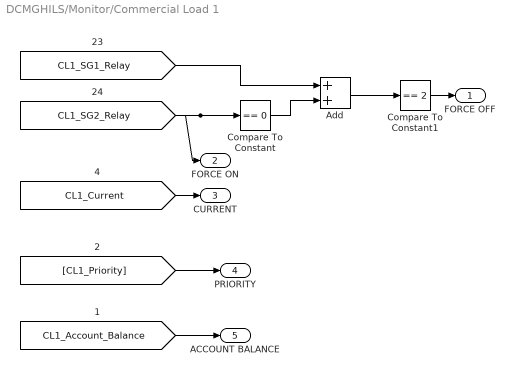
== system DCMGHILS/Monitor/Commercial Load 1 ==
  Add : Sum
  Compare To Constant : simulink/Logic and Bit Operations/Compare To Constant  relop===  const=0  OutDataTypeStr=uint8
  Compare To Constant1 : simulink/Logic and Bit Operations/Compare To Constant  relop===  const=2  OutDataTypeStr=uint8
  FORCE OFF : Outport
  FORCE ON : Outport  Port=2
  CURRENT : Outport  Port=3
  PRIORITY : Outport  Port=4
  ACCOUNT BALANCE : Outport  Port=5
  wires:
  [CL1_SG2_Relay] -> Compare To Constant/1, FORCE ON/1
  [CL1_SG1_Relay] -> Add/1
  Compare To Constant/1 -> Add/2
  Add/1 -> Compare To Constant1/1
  Compare To Constant1/1 -> FORCE OFF/1
  [CL1_Current] -> CURRENT/1
  [CL1_Priority] -> PRIORITY/1
  [CL1_Account_Balance] -> ACCOUNT BALANCE/1

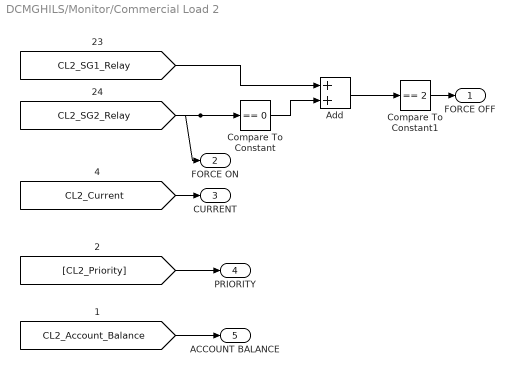
== system DCMGHILS/Monitor/Commercial Load 2 ==
  Add : Sum
  Compare To Constant : simulink/Logic and Bit Operations/Compare To Constant  relop===  const=0  OutDataTypeStr=uint8
  Compare To Constant1 : simulink/Logic and Bit Operations/Compare To Constant  relop===  const=2  OutDataTypeStr=uint8
  FORCE OFF : Outport
  FORCE ON : Outport  Port=2
  CURRENT : Outport  Port=3
  PRIORITY : Outport  Port=4
  ACCOUNT BALANCE : Outport  Port=5
  wires:
  [CL2_SG2_Relay] -> Compare To Constant/1, FORCE ON/1
  [CL2_SG1_Relay] -> Add/1
  Compare To Constant/1 -> Add/2
  Add/1 -> Compare To Constant1/1
  Compare To Constant1/1 -> FORCE OFF/1
  [CL2_Current] -> CURRENT/1
  [CL2_Priority] -> PRIORITY/1
  [CL2_Account_Balance] -> ACCOUNT BALANCE/1

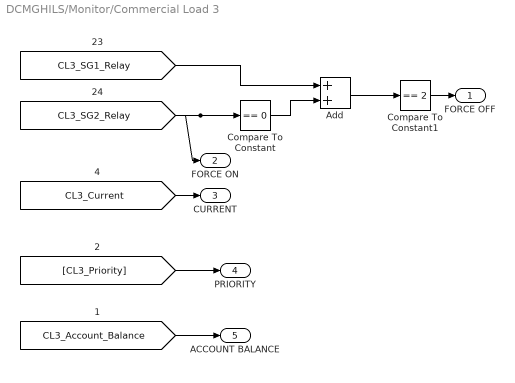
== system DCMGHILS/Monitor/Commercial Load 3 ==
  Add : Sum
  Compare To Constant : simulink/Logic and Bit Operations/Compare To Constant  relop===  const=0  OutDataTypeStr=uint8
  Compare To Constant1 : simulink/Logic and Bit Operations/Compare To Constant  relop===  const=2  OutDataTypeStr=uint8
  FORCE OFF : Outport
  FORCE ON : Outport  Port=2
  CURRENT : Outport  Port=3
  PRIORITY : Outport  Port=4
  ACCOUNT BALANCE : Outport  Port=5
  wires:
  [CL3_SG2_Relay] -> Compare To Constant/1, FORCE ON/1
  [CL3_SG1_Relay] -> Add/1
  Compare To Constant/1 -> Add/2
  Add/1 -> Compare To Constant1/1
  Compare To Constant1/1 -> FORCE OFF/1
  [CL3_Current] -> CURRENT/1
  [CL3_Priority] -> PRIORITY/1
  [CL3_Account_Balance] -> ACCOUNT BALANCE/1

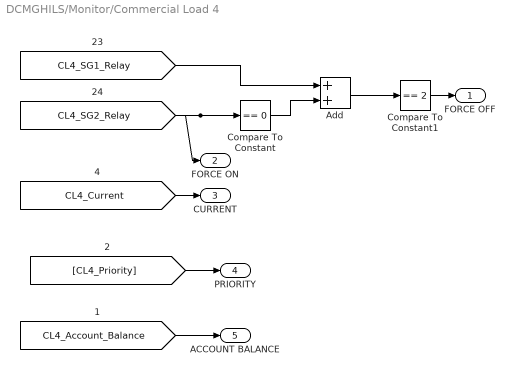
== system DCMGHILS/Monitor/Commercial Load 4 ==
  Add : Sum
  Compare To Constant : simulink/Logic and Bit Operations/Compare To Constant  relop===  const=0  OutDataTypeStr=uint8
  Compare To Constant1 : simulink/Logic and Bit Operations/Compare To Constant  relop===  const=2  OutDataTypeStr=uint8
  FORCE OFF : Outport
  FORCE ON : Outport  Port=2
  CURRENT : Outport  Port=3
  PRIORITY : Outport  Port=4
  ACCOUNT BALANCE : Outport  Port=5
  wires:
  [CL4_SG2_Relay] -> Compare To Constant/1, FORCE ON/1
  [CL4_SG1_Relay] -> Add/1
  Compare To Constant/1 -> Add/2
  Add/1 -> Compare To Constant1/1
  Compare To Constant1/1 -> FORCE OFF/1
  [CL4_Current] -> CURRENT/1
  [CL4_Priority] -> PRIORITY/1
  [CL4_Account_Balance] -> ACCOUNT BALANCE/1

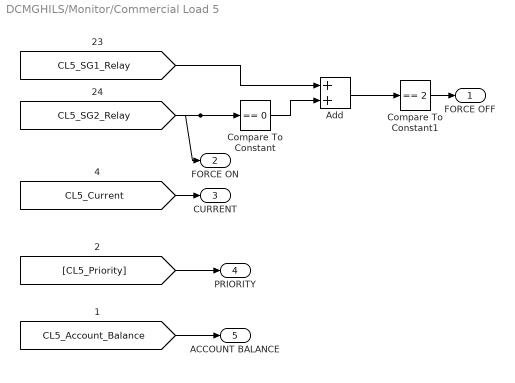
== system DCMGHILS/Monitor/Commercial Load 5 ==
  Add : Sum
  Compare To Constant : simulink/Logic and Bit Operations/Compare To Constant  relop===  const=0  OutDataTypeStr=uint8
  Compare To Constant1 : simulink/Logic and Bit Operations/Compare To Constant  relop===  const=2  OutDataTypeStr=uint8
  FORCE OFF : Outport
  FORCE ON : Outport  Port=2
  CURRENT : Outport  Port=3
  PRIORITY : Outport  Port=4
  ACCOUNT BALANCE : Outport  Port=5
  wires:
  [CL5_SG2_Relay] -> Compare To Constant/1, FORCE ON/1
  [CL5_SG1_Relay] -> Add/1
  Compare To Constant/1 -> Add/2
  Add/1 -> Compare To Constant1/1
  Compare To Constant1/1 -> FORCE OFF/1
  [CL5_Current] -> CURRENT/1
  [CL5_Priority] -> PRIORITY/1
  [CL5_Account_Balance] -> ACCOUNT BALANCE/1

== system DCMGHILS/Monitor/Grid ==
  DL_CURRENT : Outport
  DL_VOLTAGE : Outport  Port=2
  Electricity Price : Outport  Port=3
  wires:
  [DL_Current] -> DL_CURRENT/1
  [DL_Voltage] -> DL_VOLTAGE/1
  [Electricity_Price] -> Electricity Price/1

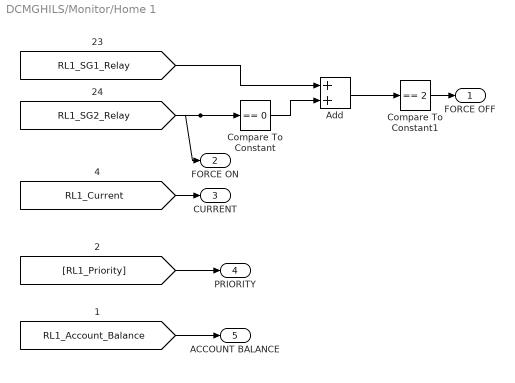
== system DCMGHILS/Monitor/Home 1 ==
  Add : Sum
  Compare To Constant : simulink/Logic and Bit Operations/Compare To Constant  relop===  const=0  OutDataTypeStr=uint8
  Compare To Constant1 : simulink/Logic and Bit Operations/Compare To Constant  relop===  const=2  OutDataTypeStr=uint8
  FORCE OFF : Outport
  FORCE ON : Outport  Port=2
  CURRENT : Outport  Port=3
  PRIORITY : Outport  Port=4
  ACCOUNT BALANCE : Outport  Port=5
  wires:
  [RL1_SG2_Relay] -> Compare To Constant/1, FORCE ON/1
  [RL1_SG1_Relay] -> Add/1
  Compare To Constant/1 -> Add/2
  Add/1 -> Compare To Constant1/1
  Compare To Constant1/1 -> FORCE OFF/1
  [RL1_Current] -> CURRENT/1
  [RL1_Priority] -> PRIORITY/1
  [RL1_Account_Balance] -> ACCOUNT BALANCE/1

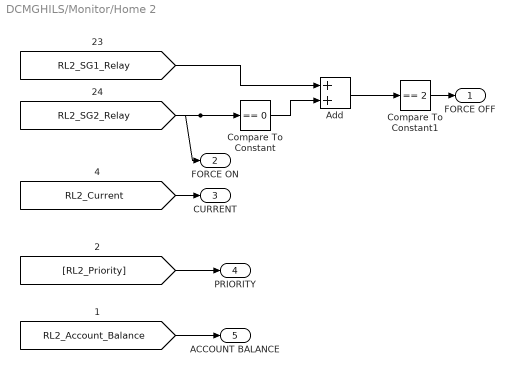
== system DCMGHILS/Monitor/Home 2 ==
  Add : Sum
  Compare To Constant : simulink/Logic and Bit Operations/Compare To Constant  relop===  const=0  OutDataTypeStr=uint8
  Compare To Constant1 : simulink/Logic and Bit Operations/Compare To Constant  relop===  const=2  OutDataTypeStr=uint8
  FORCE OFF : Outport
  FORCE ON : Outport  Port=2
  CURRENT : Outport  Port=3
  PRIORITY : Outport  Port=4
  ACCOUNT BALANCE : Outport  Port=5
  wires:
  [RL2_SG2_Relay] -> Compare To Constant/1, FORCE ON/1
  [RL2_SG1_Relay] -> Add/1
  Compare To Constant/1 -> Add/2
  Add/1 -> Compare To Constant1/1
  Compare To Constant1/1 -> FORCE OFF/1
  [RL2_Current] -> CURRENT/1
  [RL2_Priority] -> PRIORITY/1
  [RL2_Account_Balance] -> ACCOUNT BALANCE/1

== system DCMGHILS/Monitor/Home 3 ==
  Add : Sum
  Compare To Constant : simulink/Logic and Bit Operations/Compare To Constant  relop===  const=0  OutDataTypeStr=uint8
  Compare To Constant1 : simulink/Logic and Bit Operations/Compare To Constant  relop===  const=2  OutDataTypeStr=uint8
  FORCE OFF : Outport
  FORCE ON : Outport  Port=2
  CURRENT : Outport  Port=3
  PRIORITY : Outport  Port=4
  ACCOUNT BALANCE : Outport  Port=5
  wires:
  [RL3_SG2_Relay] -> Compare To Constant/1, FORCE ON/1
  [RL3_SG1_Relay] -> Add/1
  Compare To Constant/1 -> Add/2
  Add/1 -> Compare To Constant1/1
  Compare To Constant1/1 -> FORCE OFF/1
  [RL3_Current] -> CURRENT/1
  [RL3_Priority] -> PRIORITY/1
  [RL3_Account_Balance] -> ACCOUNT BALANCE/1

== system DCMGHILS/Monitor/Home 4 ==
  Add : Sum
  Compare To Constant : simulink/Logic and Bit Operations/Compare To Constant  relop===  const=0  OutDataTypeStr=uint8
  Compare To Constant1 : simulink/Logic and Bit Operations/Compare To Constant  relop===  const=2  OutDataTypeStr=uint8
  FORCE OFF : Outport
  FORCE ON : Outport  Port=2
  CURRENT : Outport  Port=3
  PRIORITY : Outport  Port=4
  ACCOUNT BALANCE : Outport  Port=5
  wires:
  [RL4_SG2_Relay] -> Compare To Constant/1, FORCE ON/1
  [RL4_SG1_Relay] -> Add/1
  Compare To Constant/1 -> Add/2
  Add/1 -> Compare To Constant1/1
  Compare To Constant1/1 -> FORCE OFF/1
  [RL4_Current] -> CURRENT/1
  [RL4_Priority] -> PRIORITY/1
  [RL4_Account_Balance] -> ACCOUNT BALANCE/1

== system DCMGHILS/Monitor/Home 5 ==
  Add : Sum
  Compare To Constant : simulink/Logic and Bit Operations/Compare To Constant  relop===  const=0  OutDataTypeStr=uint8
  Compare To Constant1 : simulink/Logic and Bit Operations/Compare To Constant  relop===  const=2  OutDataTypeStr=uint8
  FORCE OFF : Outport
  FORCE ON : Outport  Port=2
  CURRENT : Outport  Port=3
  PRIORITY : Outport  Port=4
  ACCOUNT BALANCE : Outport  Port=5
  wires:
  [RL5_SG2_Relay] -> Compare To Constant/1, FORCE ON/1
  [RL5_SG1_Relay] -> Add/1
  Compare To Constant/1 -> Add/2
  Add/1 -> Compare To Constant1/1
  Compare To Constant1/1 -> FORCE OFF/1
  [RL5_Current] -> CURRENT/1
  [RL5_Priority] -> PRIORITY/1
  [RL5_Account_Balance] -> ACCOUNT BALANCE/1

== system DCMGHILS/Monitor/Residential Branch ==
  Add : Sum
  Compare To Constant : simulink/Logic and Bit Operations/Compare To Constant  relop===  const=0  OutDataTypeStr=uint8
  Compare To Constant1 : simulink/Logic and Bit Operations/Compare To Constant  relop===  const=2  OutDataTypeStr=uint8
  FORCE OFF : Outport
  FORCE ON : Outport  Port=2
  CURRENT : Outport  Port=3
  VOLTAGE : Outport  Port=4
  wires:
  [RB_SG2_Relay] -> Compare To Constant/1, FORCE ON/1
  [RB_SG1_Relay] -> Add/1
  Compare To Constant/1 -> Add/2
  Add/1 -> Compare To Constant1/1
  Compare To Constant1/1 -> FORCE OFF/1
  [RB_Current] -> CURRENT/1
  [RB_Voltage] -> VOLTAGE/1

== system DCMGHILS/Monitor/SP ==
  FORCE OFF : Outport
  SP_CURRENT : Outport  Port=2
  SP_VOLTAGE : Outport  Port=3
  wires:
  [SP_SG_Relay] -> FORCE OFF/1
  [SP_Current] -> SP_CURRENT/1
  [SP_Voltage] -> SP_VOLTAGE/1
